simulink model "Lab4"  (R2019b)
settings: Solver=VariableStepAuto  StartTime=0.0  StopTime=10.0  RelTol=1e-3
settings Model: Creator=adity  LastModifiedBy=adity

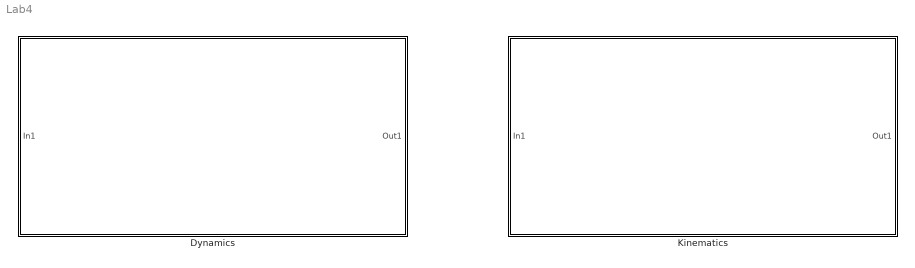
== system Lab4 ==
  Dynamics : Subsystem
  Kinematics : Subsystem

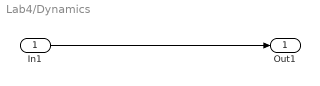
== system Lab4/Dynamics ==
  In1 : Inport
  Out1 : Outport
  wires:
  In1/1 -> Out1/1

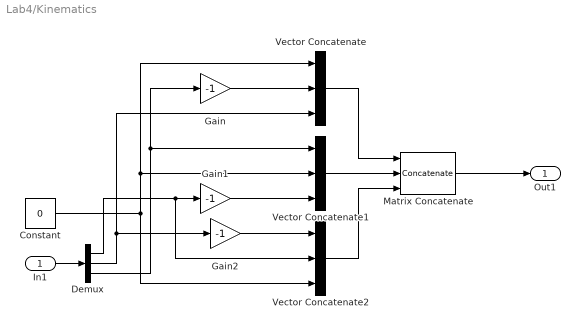
== system Lab4/Kinematics ==
  In1 : Inport
  Constant : Constant  Value=0
  Demux : Demux  Outputs=3
  Gain : Gain  Gain=-1
  Gain1 : Gain  Gain=-1
  Gain2 : Gain  Gain=-1
  Matrix Concatenate : Concatenate  NumInputs=3  Mode=Multidimensional array  ConcatenateDimension=2
  Vector Concatenate : Concatenate  NumInputs=3
  Vector Concatenate1 : Concatenate  NumInputs=3
  Vector Concatenate2 : Concatenate  NumInputs=3
  Out1 : Outport
  wires:
  In1/1 -> Demux/1
  Demux/2 -> Vector Concatenate/3, Gain2/1
  Constant/1 -> Vector Concatenate2/3, Vector Concatenate1/2, Vector Concatenate/1
  Demux/3 -> Vector Concatenate1/1, Gain/1
  Gain1/1 -> Vector Concatenate1/3
  Demux/1 -> Vector Concatenate2/2, Gain1/1
  Gain2/1 -> Vector Concatenate2/1
  Gain/1 -> Vector Concatenate/2
  Vector Concatenate/1 -> Matrix Concatenate/1
  Vector Concatenate1/1 -> Matrix Concatenate/2
  Vector Concatenate2/1 -> Matrix Concatenate/3
  Matrix Concatenate/1 -> Out1/1
